simulink model "dc_motor_exc_R2018a"  (R2018a)
settings: Solver=VariableStepAuto  StartTime=0.0  StopTime=20  RelTol=1e-3
settings Model: Creator=kjartan  LastModifiedBy=kjartan
settings DataIOCC: ReturnWorkspaceOutputs=on
settings SFSimCC: SimUseLocalCustomCode=on
settings RTWCC: RTWUseLocalCustomCode=on

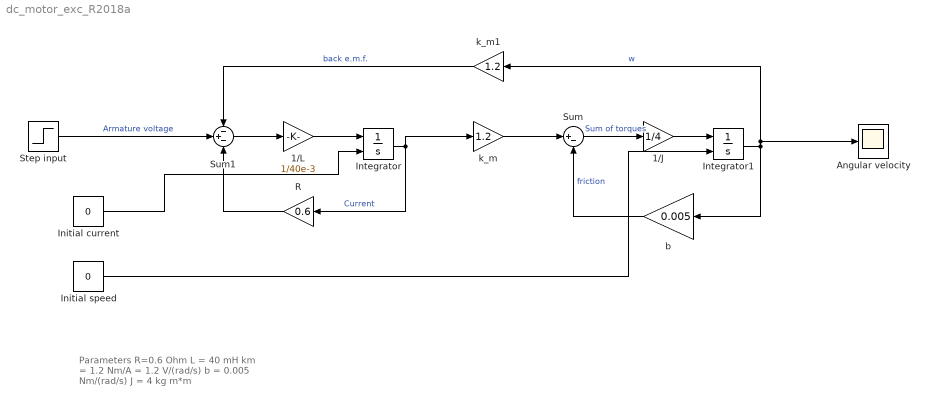
== system dc_motor_exc_R2018a ==
  note: Parameters
      |
      | R=0.6 Ohm
      | L = 40 mH
      | km = 1.2 Nm/A = 1.2 V/(rad/s)
      | b = 0.005 Nm/(rad/s)
      | J = 4 kg m*m
  1/J : Gain  Gain=1/4
  1/L : Gain  Gain=1/40e-3
  Angular velocity : Scope
  Initial current : Constant  Value=0
  Initial speed : Constant  Value=0
  Integrator : Integrator  InitialConditionSource=external
  Integrator1 : Integrator  InitialConditionSource=external
  R : Gain  Gain=0.6
  Step input : Step  After=400  SampleTime=0
  Sum : Sum  Inputs=|+-
  Sum1 : Sum  Inputs=-+-
  b : Gain  Gain=0.005
  k_m : Gain  Gain=1.2
  k_m1 : Gain  Gain=1.2
  wires:
  1/J/1 -> Integrator1/1
  Integrator1/1 -> k_m1/1, Angular velocity/1, b/1  "w"
  Sum/1 -> 1/J/1  "Sum of torques"
  b/1 -> Sum/2  "friction"
  k_m/1 -> Sum/1
  Integrator/1 -> k_m/1, R/1  "Current"
  1/L/1 -> Integrator/1
  R/1 -> Sum1/3
  Sum1/1 -> 1/L/1
  k_m1/1 -> Sum1/1  "back e.m.f."
  Step input/1 -> Sum1/2  "Armature voltage"
  Initial current/1 -> Integrator/2
  Initial speed/1 -> Integrator1/2
